simulink model "Ejer18_EcuacionesCremona"  (R2023b)
settings: Solver=FixedStepDiscrete  StartTime=0  StopTime=20  FixedStep=1  RelTol=1e-3
undefined symbols (not defined in the file): a, x1_ini, x2_ini
settings Model: Creator=alfre  LastModifiedBy=alfre

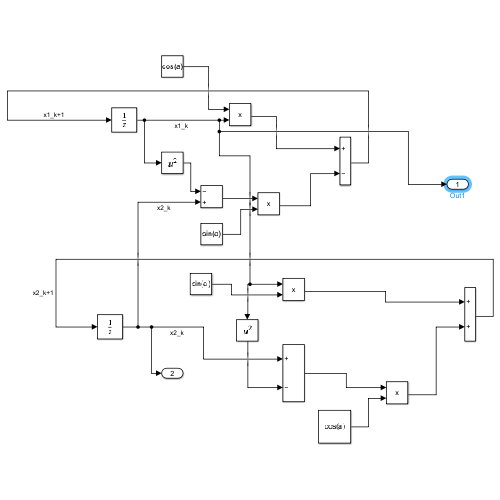
[thumbnail: Simulink's stored preview of the top-level diagram]
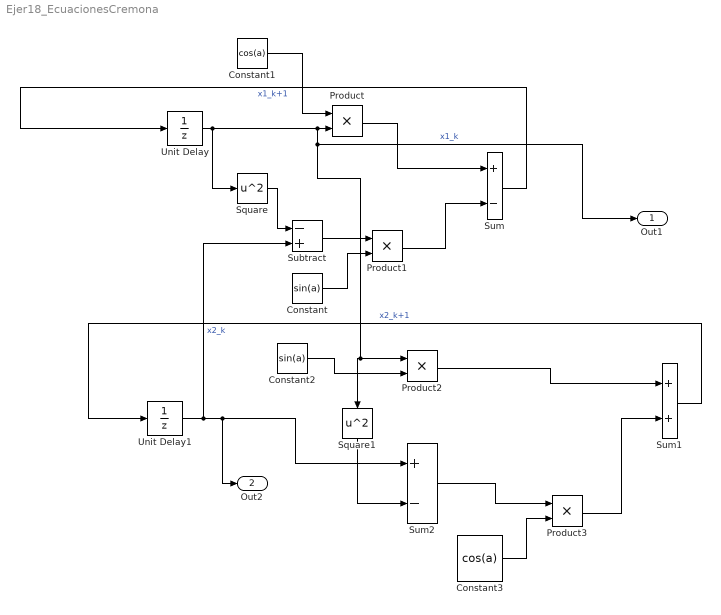
== system Ejer18_EcuacionesCremona ==
  Constant : Constant  Value=sin(a)
  Constant1 : Constant  Value=cos(a)
  Constant2 : Constant  Value=sin(a)
  Constant3 : Constant  Value=cos(a)
  Product{,1..3} (4 alike) : Product
  Square : Math  Operator=square
  Square1 : Math  Operator=square
  Subtract : Sum  Inputs=-+
  Sum : Sum  Inputs=+-
  Sum1 : Sum
  Sum2 : Sum  Inputs=+-
  Unit Delay : UnitDelay  InitialCondition=x1_ini  SampleTime=-1  HasFrameUpgradeWarning=on
  Unit Delay1 : UnitDelay  InitialCondition=x2_ini  SampleTime=-1  HasFrameUpgradeWarning=on
  Out1 : Outport
  Out2 : Outport  Port=2
  wires:
  Sum/1 -> Unit Delay/1  "x1_k+1"
  Constant1/1 -> Product/1
  Unit Delay/1 -> Square/1, Square1/1, Product2/1, Out1/1, Product/2  "x1_k"
  Product/1 -> Sum/1
  Square/1 -> Subtract/1
  Product1/1 -> Sum/2
  Subtract/1 -> Product1/1
  Constant/1 -> Product1/2
  Sum1/1 -> Unit Delay1/1  "x2_k+1"
  Unit Delay1/1 -> Subtract/2, Out2/1, Sum2/1  "x2_k"
  Constant2/1 -> Product2/2
  Product2/1 -> Sum1/1
  Square1/1 -> Sum2/2
  Sum2/1 -> Product3/1
  Constant3/1 -> Product3/2
  Product3/1 -> Sum1/2
